simulink model "LQI_sim"  (R2024b)
settings: Solver=ode5  StartTime=0.0  StopTime=tf  FixedStep=dt  RelTol=1e-3
values from neighbouring files (symbols this model uses):
  A = double(subs(jacobian(x_dot, x_vars), [x_vars;u], [x_star; u_star]))    [main_LQR.m]
  B = double(subs(jacobian(x_dot, u), [x_vars;u], [x_star; u_star]))    [main_LQR.m]
  C = [1,0,0,0; 0,0,1,0]    [main_LQR.m]
  Ki = K_aug(end)    [main_LQR.m]
  Kx = K_aug(1:4)    [main_LQR.m]
  L = place(A', C', poles_obsv)'    [main_LQR.m]
  r_pulley = 1.528*25.4/2000    (= 0.0194056)    [main_LQR.m]
  x0 = [0; 0; -9*pi/180; 0]    [main_LQR.m]
  x_star = [0;0;0;0]    [main_LQR.m]
libraries: simulink_extras x1
settings Model: Creator=johnc  LastModifiedBy=jcglenn

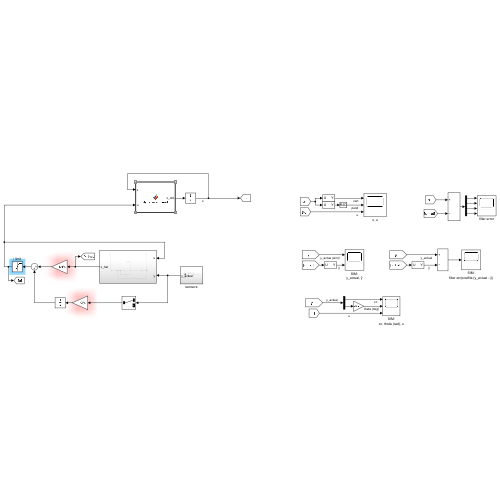
[thumbnail: Simulink's stored preview of the top-level diagram]
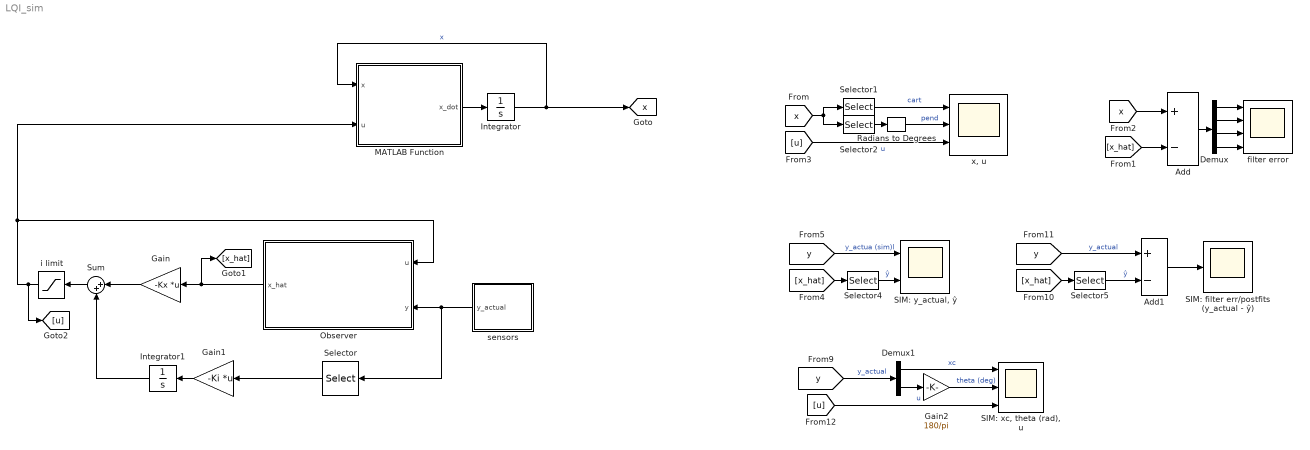
== system LQI_sim ==
  Add : Sum  Inputs=+-
  Add1 : Sum  Inputs=+-
  Demux : Demux
  Demux1 : Demux  Outputs=2
  Gain : Gain  Gain=-Kx  Multiplication=Matrix(K*u)
  Gain1 : Gain  Gain=-Ki  Multiplication=Matrix(K*u)
  Gain2 : Gain  Gain=180/pi
  Integrator : Integrator  InitialCondition=x0
  Integrator1 : Integrator
  MATLAB Function : MATLAB Function  TreatAsAtomicUnit=on
  Observer : Subsystem
  Radians to Degrees : simulink_extras/Transformations/Radians to Degrees
  SIM: filter err/postfits (y_actual - ŷ) : Scope
  "SIM: xc, theta (rad), u" : Scope  NumInputPorts=3
  "SIM: y_actual, ŷ" : Scope  NumInputPorts=2
  Selector : Selector  InputPortWidth=2  IndexOptions=Index vector (dialog)  Indices=1  OutputSizes=1
  Selector1 : Selector  InputPortWidth=4  IndexOptions=Index vector (dialog)  Indices=[1 2]  OutputSizes=1
  Selector2 : Selector  InputPortWidth=4  IndexOptions=Index vector (dialog)  Indices=[3 4]  OutputSizes=1
  Selector4 : Selector  InputPortWidth=4  IndexOptions=Index vector (dialog)  Indices=[1 3]  OutputSizes=1
  Selector5 : Selector  InputPortWidth=4  IndexOptions=Index vector (dialog)  Indices=[1 3]  OutputSizes=1
  Sum : Sum  Inputs=|++
  filter error : Scope  NumInputPorts=4
  i limit : Saturate  UpperLimit=5.1  LowerLimit=-5.1
  sensors : Subsystem
  "x, u" : Scope  NumInputPorts=3
  tag scope: x=global
  wires:
  MATLAB Function/1(x_dot) -> Integrator/1
  Integrator/1 -> [x], MATLAB Function/1(x)  "x"
  Observer/1(x_hat) -> [x_hat], Gain/1
  Gain/1 -> Sum/1
  Gain1/1 -> Integrator1/1
  Integrator1/1 -> Sum/2
  Sum/1 -> i limit/1
  i limit/1 -> Observer/1(u), MATLAB Function/2(u), [u]
  Selector4/1 -> "SIM: y_actual, ŷ"/2  "ŷ"
  [x_hat] -> Add/2
  Demux/3 -> filter error/3
  Add/1 -> Demux/1
  Demux/2 -> filter error/2
  [x] -> Add/1
  Demux1/1 -> "SIM: xc, theta (rad), u"/1  "xc"
  [y] -> Demux1/1  "y_actual"
  Demux/1 -> filter error/1
  [x_hat] -> Selector5/1
  Radians to Degrees/1 -> "x, u"/2  "pend"
  Selector2/1 -> Radians to Degrees/1
  [u] -> "SIM: xc, theta (rad), u"/3  "u"
  [x_hat] -> Selector4/1
  Selector1/1 -> "x, u"/1  "cart"
  Selector5/1 -> Add1/2  "ŷ"
  [y] -> "SIM: y_actual, ŷ"/1  "y_actua (sim)l"
  [y] -> Add1/1  "y_actual"
  Gain2/1 -> "SIM: xc, theta (rad), u"/2  "theta (deg)"
  [x] -> Selector1/1, Selector2/1
  Demux1/2 -> Gain2/1
  Add1/1 -> SIM: filter err/postfits (y_actual - ŷ)/1
  Demux/4 -> filter error/4
  [u] -> "x, u"/3  "u"
  Selector/1 -> Gain1/1
  sensors/1(y_actual) -> Selector/1, Observer/2(y)

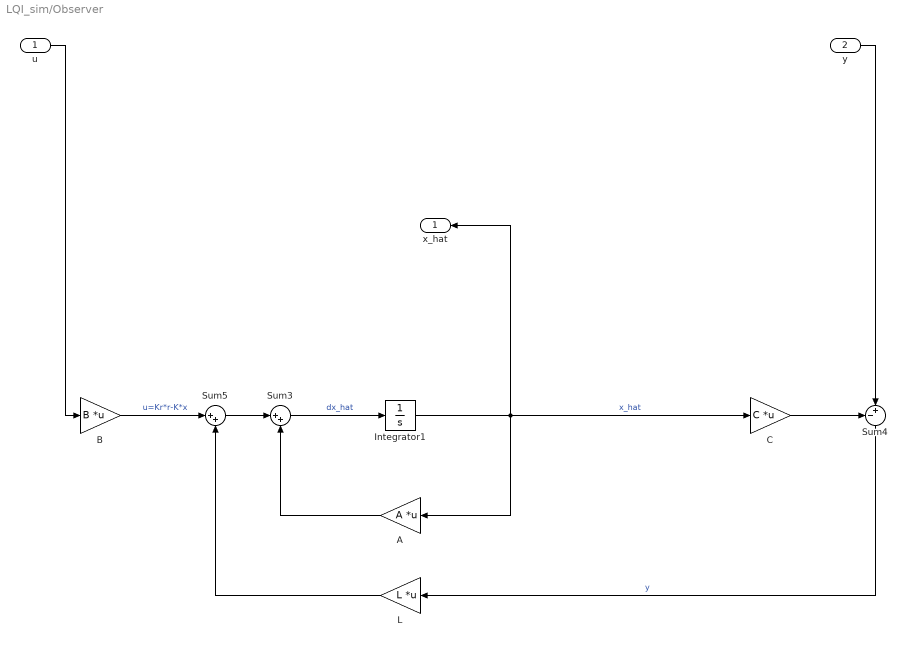
== system LQI_sim/Observer ==
  u : Inport
  y : Inport  Port=2
  A : Gain  Gain=A  Multiplication=Matrix(K*u)
  B : Gain  Gain=B  Multiplication=Matrix(K*u)
  C : Gain  Gain=C  Multiplication=Matrix(K*u)
  Integrator1 : Integrator  InitialCondition=x0-x_star
  L : Gain  Gain=L  Multiplication=Matrix(K*u)
  Sum3 : Sum  Inputs=|++
  Sum4 : Sum  Inputs=-+|
  Sum5 : Sum  Inputs=|++
  x_hat : Outport
  wires:
  C/1 -> Sum4/1
  Integrator1/1 -> x_hat/1, C/1, A/1  "x_hat"
  Sum5/1 -> Sum3/1
  L/1 -> Sum5/2
  A/1 -> Sum3/2
  Sum4/1 -> L/1  "y"
  Sum3/1 -> Integrator1/1  "dx_hat"
  B/1 -> Sum5/1  "u=Kr*r-K*x"
  u/1 -> B/1
  y/1 -> Sum4/2

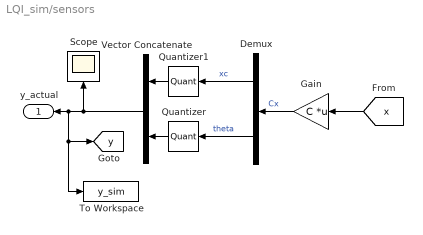
== system LQI_sim/sensors ==
  Demux : Demux  Outputs=2
  Gain : Gain  Gain=C  Multiplication=Matrix(K*u)
  Quantizer : Quantizer  QuantizationInterval=2*pi/10000
  Quantizer1 : Quantizer  QuantizationInterval=2*pi*r_pulley/10000
  Scope : Scope
  To Workspace : ToWorkspace  VariableName=y_sim  SampleTime=-1
  Vector Concatenate : Concatenate  Mode=Multidimensional array
  y_actual : Outport
  tag scope: y=global
  wires:
  Demux/1 -> Quantizer1/1  "xc"
  Demux/2 -> Quantizer/1  "theta"
  Quantizer1/1 -> Vector Concatenate/1
  Quantizer/1 -> Vector Concatenate/2
  [x] -> Gain/1
  Vector Concatenate/1 -> To Workspace/1, [y], y_actual/1, Scope/1
  Gain/1 -> Demux/1  "Cx"

== matlab function LQI_sim/MATLAB Function ==
  data: x input; x_dot output; u input; params parameter
function x_dot  = dynamics_pend(x, u, params)

g = params.g;
mc = params.mc;
mp = params.mp;
Jp = params.Jp;
bc = params.bc;
bp = params.bp;
Lp = params.Lp;
r_pulley = params.r_pulley;
Ke = params.Ke;
Fc = params.Fc;

x1 = x(1);
x2 = x(2);
x3 = x(3);
x4 = x(4);

F_fric = Fc*tanh(100*x2);
% F_fric = 0; %COMMENT OUT

x1_dot = x2;
x2_dot = (Ke*u/r_pulley - bc*x2 - F_fric - mp*Lp*x4^2*sin(x3) + mp*Lp*cos(x3)*(-bp*x4 + mp*g*Lp*sin(x3))/(mp*Lp^2 + Jp))*1/(mc + mp - mp^2*Lp^2*cos(x3)^2/(mp*Lp^2 + Jp));
x3_dot = x4;
x4_dot = (-bp*x4 + mp*g*Lp*sin(x3) + mp*Lp*cos(x3)*(Ke*u/r_pulley - bc*x2 - mp*Lp*x4^2*sin(x3))/(mc + mp))*1/(mp*Lp^2 + Jp - mp^2*Lp^2*cos(x3)^2/(mc + mp));

x_dot = [x1_dot; x2_dot; x3_dot; x4_dot];
